simulink model "QBot2e_Particle_Filtering"  (Simulink 8.9)
settings: Solver=ode1  StartTime=0.0  StopTime=inf  FixedStep=0.01  RelTol=1e-3  EnableMultiTasking=on
InitFcn:
  | p=1:640; % pixels from left to right
  | 
  | Obtained_angles=(320-p).*(57/640)*pi./180;  % Kinect's horizontal FOV = 57 degrees
undefined symbols (not defined in the file): HIL, qc_get_step_size, Video3D
libraries: quarc_library x9, simulink x5
settings Model: Creator=drmadill  LastModifiedBy=User  SimulationMode=external  ExtModeTrigDuration=2
settings SolverCC: PositivePriorityOrder=on
settings OptimizationCC: ExpressionDepthLimit=2147483647  LifeSpan=auto
settings DebuggingCC: SolverPrmCheckMsg=warning
settings RTWCC: SystemTargetFile=quarc_linux_pi_3.tlc  TemplateMakefile=quarc_linux_pi_3_tmf  Description=QUARC Linux Raspberry Pi 3 Target
settings STFCustomTargetCC: TargetLibSuffix=.a  TargetPreCompLibLocation=C:\PROGRA~3\QUARC\lib\2019b\LINUX_~1\release  ConcurrentExecutionCompliant=on  SystemTargetFile=quarc_linux_pi_3.tlc
settings GRTTargetCC: TargetLibSuffix=.a  TargetPreCompLibLocation=C:\PROGRA~3\QUARC\lib\2017a\LICFC8~1\release  ParMdlRefBuildCompliant=off  CompOptLevelCompliant=off  GeneratePreprocessorConditionals=Use local settings  MatFileLogging=off  CPPClassGenCompliant=off  UseToolchainInfoCompliant=off  ExtMode=on  ExtModeMexFile=quarc_comm  ExtModeMexArgs='-w -d /tmp -uri %u'
settings ConfigComp: CovSFcnEnable=off

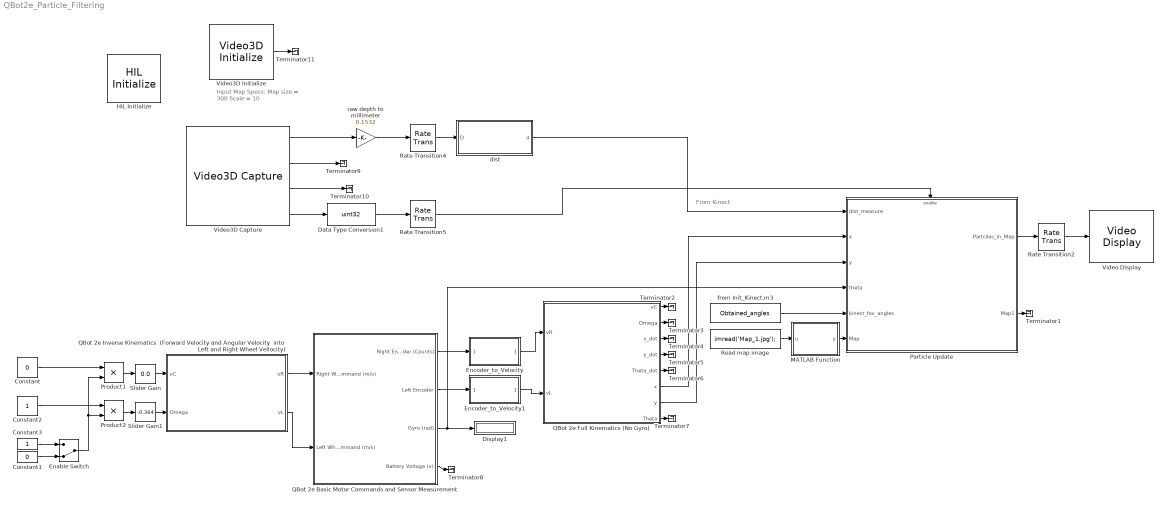
== system QBot2e_Particle_Filtering ==
  note: From Kinect
  note: Input Map Specs:
      | Map size = 300
      | Scale = 10
  Constant : Constant  Value=0
  Constant1 : Constant  Value=0
  Constant2 : Constant
  Constant3 : Constant
  Data Type Conversion1 : DataTypeConversion  OutDataTypeStr=uint32
  Display1 : Display
  Enable Switch : ManualSwitch  CurrentSetting=0
  Encoder_to_Velocity : Subsystem
  Encoder_to_Velocity1 : Subsystem
  HIL Initialize : quarc_library/Data Acquisition/Generic/Configuration/HIL Initialize  Priority=-99  object_name=HIL-1  board_type=qbot2e  board_number=0  board_options=pwm0_en=1;pwm0_pin=12;pwm1_en=1;pwm1_pin=13;  exclusive=off  active=off  hardware_clocks=[]  clock_modes=[]  initial_clock_frequencies=[]  set_clock_params_at_start=off  set_clock_params_at_switch_in=off  set_clock_frequencies_at_start=off  set_clock_frequencies_at_switch_in=off  analog_input_channels=[0:5]  analog_input_configurations=[]  analog_input_maximums=[16.5 3.3 3.3 3.3 3.3 3.3]  analog_input_minimums=[0 0 0 0 0 0]  set_analog_input_params_at_start=off  set_analog_input_params_at_switch_in=off  analog_output_channels=[]  analog_output_maximums=[]  analog_output_minimums=[]  initial_analog_outputs=[]  final_analog_outputs=[]  watchdog_analog_outputs=[]  set_analog_output_params_at_start=off  set_analog_output_params_at_switch_in=off  set_analog_outputs_at_start=off  set_analog_outputs_at_switch_in=off  set_analog_outputs_at_terminate=off  set_analog_outputs_at_switch_out=off  set_analog_outputs_on_watchdog=off  digital_input_channels=[28:58]  digital_output_channels=[28:31]  digital_output_configuration=[]  initial_digital_outputs=[0]  final_digital_outputs=[0]  watchdog_digital_outputs=[]  set_digital_output_params_at_start=off  set_digital_output_params_at_switch_in=off  set_digital_outputs_at_start=on  set_digital_outputs_at_switch_in=off  set_digital_outputs_at_terminate=on  set_digital_outputs_at_switch_out=off  set_digital_outputs_on_watchdog=off  encoder_channels=[0:1]  quadrature=[4]  encoder_filter_frequency=[]  initial_encoder_counts=[0]  set_encoder_params_at_start=on  set_encoder_params_at_switch_in=off  set_encoder_counts_at_start=on  set_encoder_counts_at_switch_in=off  pwm_channels=[0:1]  pwm_modes=0  pwm_frequency=100e6 / 4095  pwm_configuration=[0]  pwm_alignment=[0]  pwm_polarity=[1]  pwm_leading_deadband=[]  pwm_trailing_deadband=[]  initial_pwm_outputs=[0]  final_pwm_outputs=[0]  watchdog_pwm_outputs=[]  set_pwm_params_at_start=on  set_pwm_params_at_switch_in=off  set_pwm_outputs_at_start=on  set_pwm_outputs_at_switch_in=off  set_pwm_outputs_at_terminate=on  set_pwm_outputs_at_switch_out=off  set_pwm_outputs_on_watchdog=off  other_output_channels=[2000:2001 14000 16000]  initial_other_outputs=[0 0 0 7]  final_other_outputs=[0 0 0 7]  watchdog_other_outputs=[]  set_other_outputs_at_start=on  set_other_outputs_at_switch_in=off  set_other_outputs_at_terminate=on  set_other_outputs_at_switch_out=off  set_other_outputs_on_watchdog=off
  MATLAB Function : MATLAB Function  TreatAsAtomicUnit=on
  Particle Update : Subsystem  TreatAsAtomicUnit=on
  Product1 : Product  RndMeth=Zero
  Product2 : Product  RndMeth=Zero
  QBot 2e Basic Motor Commands and Sensor Measurement : Subsystem
  QBot 2e Full Kinematics (No Gyro) : Subsystem
  QBot 2e Inverse Kinematics  (Forward Velocity and Angular Velocity  into Left and Right Wheel Vellocity) : Subsystem
  Rate Transition2 : RateTransition
  Rate Transition4 : RateTransition
  Rate Transition5 : RateTransition
  Read map image : Constant  Value=imread('Map_1.jpg');
  Slider Gain : simulink/Math Operations/Slider Gain  gain=0.0  low=-1  high=1
  Slider Gain1 : simulink/Math Operations/Slider Gain  gain=-0.364  low=-0.7  high=0.7
  Terminator{1..11} (11 alike) : Terminator
  Video Display : quarc_library/Multimedia/Video Display  Tag=QBot2e_Particle_Filtering/Video Display  sample_time=-1  use_hardware=on
  Video3D Capture : quarc_library/Multimedia/Video3D Capture  object_name=Video3D-1  stream_type=Depth  stream_index=0  resolution=640 x 480  width=640  height=480  output_format=MATLAB greyscale (HxW)  data_type=uint16  sample_time=qc_get_step_size * ceil(0.033 / qc_get_step_size)  brightness_override=off  brightness=50.0  contrast_override=off  contrast=50.0  hue_override=off  hue=50.0  saturation_override=off  saturation=50.0  sharpness_override=off  sharpness=50.0  gamma_override=off  gamma=50.0  gain_override=off  gain=50.0  backlightcompensation_override=off  backlightcompensation=50.0  whitebalance_override=Automatic white balance  whitebalance=50.0  exposure_override=Automatic exposure  exposure=30.0  emitter=Enable laser emitter  preset=Do not set camera presets
  Video3D Initialize : quarc_library/Multimedia/Video3D Initialize  object_name=Video3D-1  source=Device  identifier=0  file=sample.bag  sample_time=qc_get_step_size * ceil(0.033 / qc_get_step_size)  active=on
  dist : MATLAB Function  TreatAsAtomicUnit=on
  from Init_Kinect.m3 : Constant  Value=Obtained_angles
  raw depth to millimeter : Gain  Gain=0.1532
  wires:
  Constant3/1 -> Enable Switch/1
  QBot 2e Basic Motor Commands and Sensor Measurement/1(Right Encoder (Counts)) -> Encoder_to_Velocity/1(Encoder)
  QBot 2e Basic Motor Commands and Sensor Measurement/2(Left Encoder) -> Encoder_to_Velocity1/1(Encoder)
  QBot 2e Basic Motor Commands and Sensor Measurement/3(Gyro (rad)) -> Display1/1, Particle Update/4(theta)
  QBot 2e Full Kinematics (No Gyro)/7(y) -> Particle Update/3(y)
  QBot 2e Full Kinematics (No Gyro)/6(x) -> Particle Update/2(x)
  Slider Gain/1 -> QBot 2e Inverse Kinematics  (Forward Velocity and Angular Velocity  into Left and Right Wheel Vellocity)/1(vC)
  Slider Gain1/1 -> QBot 2e Inverse Kinematics  (Forward Velocity and Angular Velocity  into Left and Right Wheel Vellocity)/2(Omega)
  from Init_Kinect.m3/1 -> Particle Update/5(kinect_fov_angles)
  dist/1(d) -> Particle Update/1(dist_measure)
  Particle Update/2(Map1) -> Terminator1/1
  QBot 2e Inverse Kinematics  (Forward Velocity and Angular Velocity  into Left and Right Wheel Vellocity)/1(vR) -> QBot 2e Basic Motor Commands and Sensor Measurement/1(Right Wheel Command (m/s))
  QBot 2e Inverse Kinematics  (Forward Velocity and Angular Velocity  into Left and Right Wheel Vellocity)/2(vL) -> QBot 2e Basic Motor Commands and Sensor Measurement/2(Left Wheel Command (m/s))
  Product1/1 -> Slider Gain/1
  Product2/1 -> Slider Gain1/1
  Enable Switch/1 -> Product2/2, Product1/2
  Constant/1 -> Product1/1
  Constant2/1 -> Product2/1
  Encoder_to_Velocity/1(Velocity) -> QBot 2e Full Kinematics (No Gyro)/1(vR)
  Encoder_to_Velocity1/1(Velocity) -> QBot 2e Full Kinematics (No Gyro)/2(vL)
  Constant1/1 -> Enable Switch/2
  QBot 2e Full Kinematics (No Gyro)/1(vC) -> Terminator2/1
  QBot 2e Full Kinematics (No Gyro)/2(Omega) -> Terminator3/1
  QBot 2e Full Kinematics (No Gyro)/3(x_dot) -> Terminator4/1
  QBot 2e Full Kinematics (No Gyro)/4(y_dot) -> Terminator5/1
  QBot 2e Full Kinematics (No Gyro)/5(Theta_dot) -> Terminator6/1
  QBot 2e Full Kinematics (No Gyro)/8(Theta) -> Terminator7/1
  Particle Update/1(Partciles_in_Map) -> Rate Transition2/1
  Rate Transition2/1 -> Video Display/1
  Read map image/1 -> MATLAB Function/1(u)
  MATLAB Function/1(y) -> Particle Update/6(Map)
  QBot 2e Basic Motor Commands and Sensor Measurement/4(Battery Voltage (v)) -> Terminator8/1
  Video3D Capture/2 -> Terminator9/1
  Video3D Capture/3 -> Terminator10/1
  Video3D Initialize/1 -> Terminator11/1
  Rate Transition5/1 -> Particle Update/Enable
  Video3D Capture/1 -> raw depth to millimeter/1
  Video3D Capture/4 -> Data Type Conversion1/1
  Data Type Conversion1/1 -> Rate Transition5/1
  Rate Transition4/1 -> dist/1(D)
  raw depth to millimeter/1 -> Rate Transition4/1

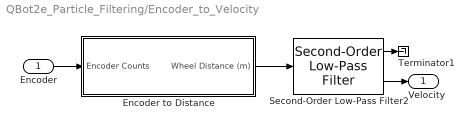
== system QBot2e_Particle_Filtering/Encoder_to_Velocity ==
  Encoder : Inport
  Encoder to Distance : Subsystem
  Second-Order Low-Pass Filter2 : quarc_library/Continuous/Second-Order Low-Pass Filter  params_source=Internal (dialog parameters)  input_width=10  input_zeta=1  input_init=0
  Terminator1 : Terminator
  Velocity : Outport
  wires:
  Second-Order Low-Pass Filter2/1 -> Terminator1/1
  Encoder to Distance/1(Wheel Distance (m)) -> Second-Order Low-Pass Filter2/1
  Encoder/1 -> Encoder to Distance/1(Encoder Counts)
  Second-Order Low-Pass Filter2/2 -> Velocity/1

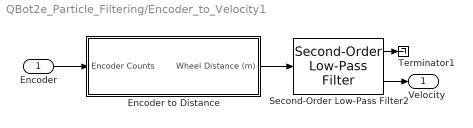
== system QBot2e_Particle_Filtering/Encoder_to_Velocity1 ==
  Encoder : Inport
  Encoder to Distance : Subsystem
  Second-Order Low-Pass Filter2 : quarc_library/Continuous/Second-Order Low-Pass Filter  params_source=Internal (dialog parameters)  input_width=10  input_zeta=1  input_init=0
  Terminator1 : Terminator
  Velocity : Outport
  wires:
  Second-Order Low-Pass Filter2/1 -> Terminator1/1
  Encoder to Distance/1(Wheel Distance (m)) -> Second-Order Low-Pass Filter2/1
  Encoder/1 -> Encoder to Distance/1(Encoder Counts)
  Second-Order Low-Pass Filter2/2 -> Velocity/1

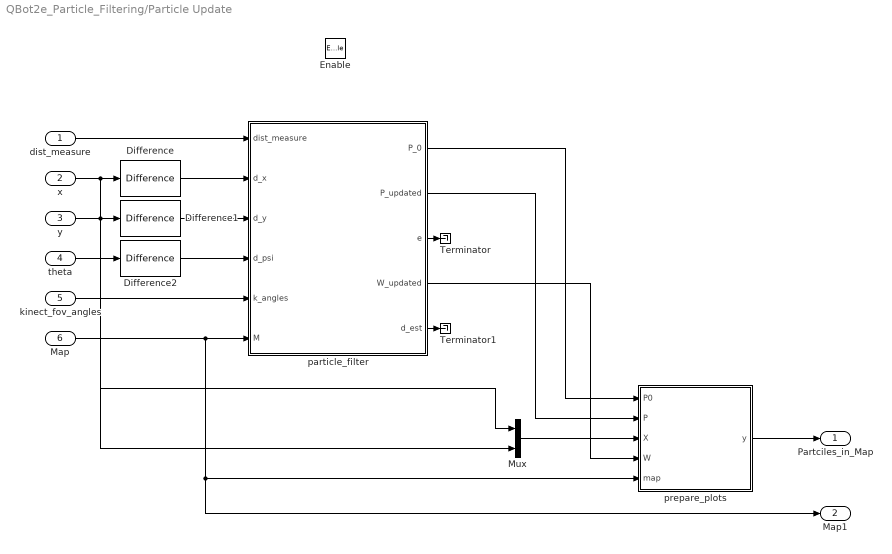
== system QBot2e_Particle_Filtering/Particle Update ==
  dist_measure : Inport
  x : Inport  Port=2
  y : Inport  Port=3
  theta : Inport  Port=4
  kinect_fov_angles : Inport  Port=5
  Map : Inport  Port=6
  Enable : EnablePort
  Difference : simulink/Discrete/Difference  ICPrevInput=0.0  OutMin=[]  OutMax=[]  OutDataType=fixdt(1, 16)  OutScaling=2^-10  DoSatur=off
  Difference1 : simulink/Discrete/Difference  ICPrevInput=0.0  OutMin=[]  OutMax=[]  OutDataType=fixdt(1, 16)  OutScaling=2^-10  DoSatur=off
  Difference2 : simulink/Discrete/Difference  ICPrevInput=0.0  OutMin=[]  OutMax=[]  OutDataType=fixdt(1, 16)  OutScaling=2^-10  DoSatur=off
  Mux : Mux  Inputs=2
  Terminator : Terminator
  Terminator1 : Terminator
  particle_filter : MATLAB Function  TreatAsAtomicUnit=on
  prepare_plots : MATLAB Function  TreatAsAtomicUnit=on
  Partciles_in_Map : Outport
  Map1 : Outport  Port=2
  wires:
  Map/1 -> Map1/1, prepare_plots/5(map), particle_filter/6(M)
  theta/1 -> Difference2/1
  y/1 -> Mux/2, Difference1/1
  x/1 -> Mux/1, Difference/1
  particle_filter/4(W_updated) -> prepare_plots/4(W)
  Difference2/1 -> particle_filter/4(d_psi)
  Difference1/1 -> particle_filter/3(d_y)
  Difference/1 -> particle_filter/2(d_x)
  Mux/1 -> prepare_plots/3(X)
  prepare_plots/1(y) -> Partciles_in_Map/1
  particle_filter/1(P_0) -> prepare_plots/1(P0)
  kinect_fov_angles/1 -> particle_filter/5(k_angles)
  particle_filter/2(P_updated) -> prepare_plots/2(P)
  dist_measure/1 -> particle_filter/1(dist_measure)
  particle_filter/3(e) -> Terminator/1
  particle_filter/5(d_est) -> Terminator1/1

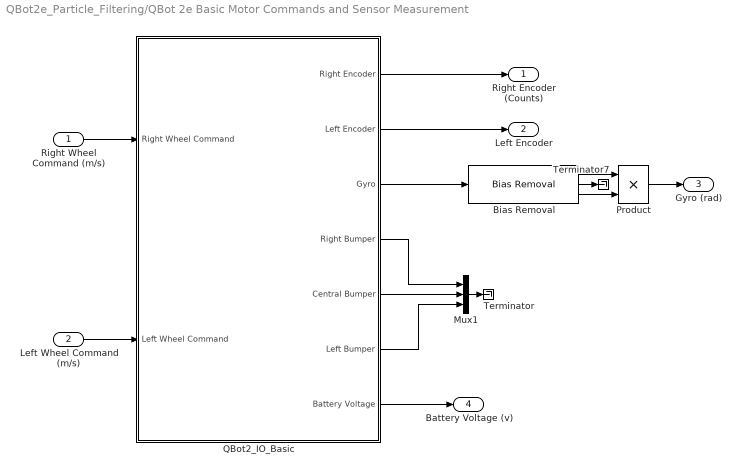
== system QBot2e_Particle_Filtering/QBot 2e Basic Motor Commands and Sensor Measurement ==
  Right Wheel Command (m/s) : Inport
  Left Wheel Command (m/s) : Inport  Port=2
  Bias Removal : quarc_library/Discrete/Bias Removal  start_time=3  end_time=4  switch_id=0  sample_time=qc_get_step_size
      settings: SourceProductName=QUARC Targets
  Mux1 : Mux  Inputs=3
  Product : Product  RndMeth=Zero
  QBot2_IO_Basic : Subsystem
  Terminator : Terminator
  Terminator7 : Terminator
  Right Encoder (Counts) : Outport
  Left Encoder : Outport  Port=2
  Gyro (rad) : Outport  Port=3
  Battery Voltage (v) : Outport  Port=4
  wires:
  QBot2_IO_Basic/4(Right Bumper) -> Mux1/1
  QBot2_IO_Basic/5(Central Bumper) -> Mux1/2
  QBot2_IO_Basic/6(Left Bumper) -> Mux1/3
  Right Wheel Command (m/s)/1 -> QBot2_IO_Basic/1(Right Wheel Command)
  Left Wheel Command (m/s)/1 -> QBot2_IO_Basic/2(Left Wheel Command)
  QBot2_IO_Basic/1(Right Encoder) -> Right Encoder (Counts)/1
  QBot2_IO_Basic/2(Left Encoder) -> Left Encoder/1
  QBot2_IO_Basic/7(Battery Voltage) -> Battery Voltage (v)/1
  Bias Removal/2 -> Terminator7/1
  Bias Removal/1 -> Product/1
  Bias Removal/3 -> Product/2
  Product/1 -> Gyro (rad)/1
  QBot2_IO_Basic/3(Gyro) -> Bias Removal/1
  Mux1/1 -> Terminator/1

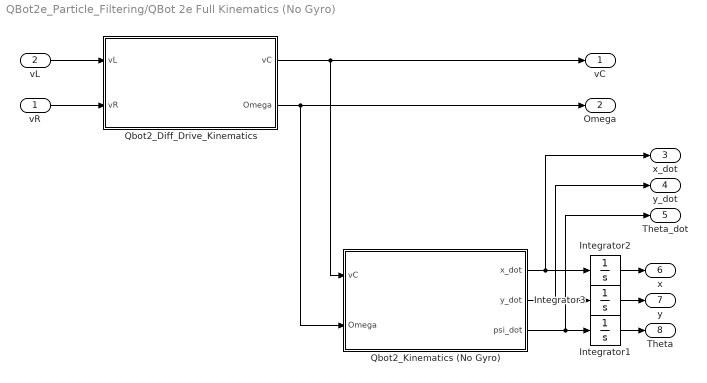
== system QBot2e_Particle_Filtering/QBot 2e Full Kinematics (No Gyro) ==
  vR : Inport
  vL : Inport  Port=2
  Integrator1 : Integrator
  Integrator2 : Integrator
  Integrator3 : Integrator
  Qbot2_Diff_Drive_Kinematics : Subsystem
  Qbot2_Kinematics (No Gyro) : Subsystem
  vC : Outport
  Omega : Outport  Port=2
  x_dot : Outport  Port=3
  y_dot : Outport  Port=4
  Theta_dot : Outport  Port=5
  x : Outport  Port=6
  y : Outport  Port=7
  Theta : Outport  Port=8
  wires:
  Qbot2_Diff_Drive_Kinematics/2(Omega) -> Omega/1, Qbot2_Kinematics (No Gyro)/2(Omega)
  Integrator3/1 -> y/1
  Integrator2/1 -> x/1
  vR/1 -> Qbot2_Diff_Drive_Kinematics/2(vR)
  vL/1 -> Qbot2_Diff_Drive_Kinematics/1(vL)
  Qbot2_Diff_Drive_Kinematics/1(vC) -> vC/1, Qbot2_Kinematics (No Gyro)/1(vC)
  Qbot2_Kinematics (No Gyro)/2(y_dot) -> Integrator3/1, y_dot/1
  Qbot2_Kinematics (No Gyro)/1(x_dot) -> Integrator2/1, x_dot/1
  Qbot2_Kinematics (No Gyro)/3(psi_dot) -> Integrator1/1, Theta_dot/1
  Integrator1/1 -> Theta/1

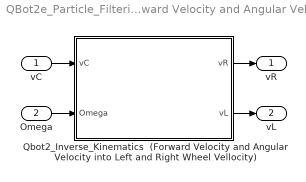
== system QBot2e_Particle_Filtering/QBot 2e Inverse Kinematics  (Forward Velocity and Angular Velocity  into Left and Right Wheel Vellocity) ==
  vC : Inport
  Omega : Inport  Port=2
  Qbot2_Inverse_Kinematics  (Forward Velocity and Angular Velocity into Left and Right Wheel Vellocity) : MATLAB Function  TreatAsAtomicUnit=on
  vR : Outport
  vL : Outport  Port=2
  wires:
  vC/1 -> Qbot2_Inverse_Kinematics  (Forward Velocity and Angular Velocity into Left and Right Wheel Vellocity)/1(vC)
  Qbot2_Inverse_Kinematics  (Forward Velocity and Angular Velocity into Left and Right Wheel Vellocity)/1(vR) -> vR/1
  Omega/1 -> Qbot2_Inverse_Kinematics  (Forward Velocity and Angular Velocity into Left and Right Wheel Vellocity)/2(Omega)
  Qbot2_Inverse_Kinematics  (Forward Velocity and Angular Velocity into Left and Right Wheel Vellocity)/2(vL) -> vL/1

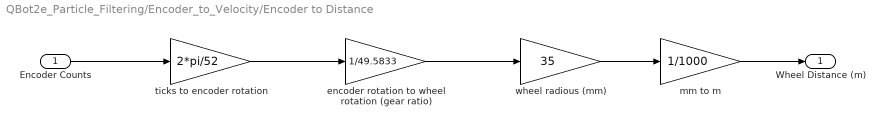
== system QBot2e_Particle_Filtering/Encoder_to_Velocity/Encoder to Distance ==
  Encoder Counts : Inport
  " encoder rotation to wheel rotation (gear ratio)" : Gain  Gain=1/49.5833
  mm to m : Gain  Gain=1/1000
  ticks to encoder rotation : Gain  Gain=2*pi/52
  wheel radious (mm) : Gain  Gain=35
  Wheel Distance (m) : Outport
  wires:
  Encoder Counts/1 -> ticks to encoder rotation/1
  ticks to encoder rotation/1 -> " encoder rotation to wheel rotation (gear ratio)"/1
  " encoder rotation to wheel rotation (gear ratio)"/1 -> wheel radious (mm)/1
  wheel radious (mm)/1 -> mm to m/1
  mm to m/1 -> Wheel Distance (m)/1

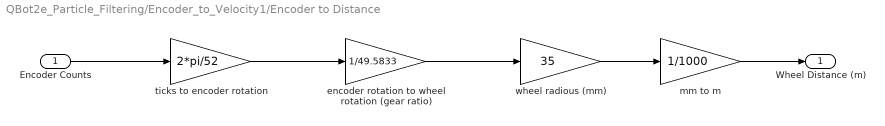
== system QBot2e_Particle_Filtering/Encoder_to_Velocity1/Encoder to Distance ==
  Encoder Counts : Inport
  " encoder rotation to wheel rotation (gear ratio)" : Gain  Gain=1/49.5833
  mm to m : Gain  Gain=1/1000
  ticks to encoder rotation : Gain  Gain=2*pi/52
  wheel radious (mm) : Gain  Gain=35
  Wheel Distance (m) : Outport
  wires:
  Encoder Counts/1 -> ticks to encoder rotation/1
  ticks to encoder rotation/1 -> " encoder rotation to wheel rotation (gear ratio)"/1
  " encoder rotation to wheel rotation (gear ratio)"/1 -> wheel radious (mm)/1
  wheel radious (mm)/1 -> mm to m/1
  mm to m/1 -> Wheel Distance (m)/1

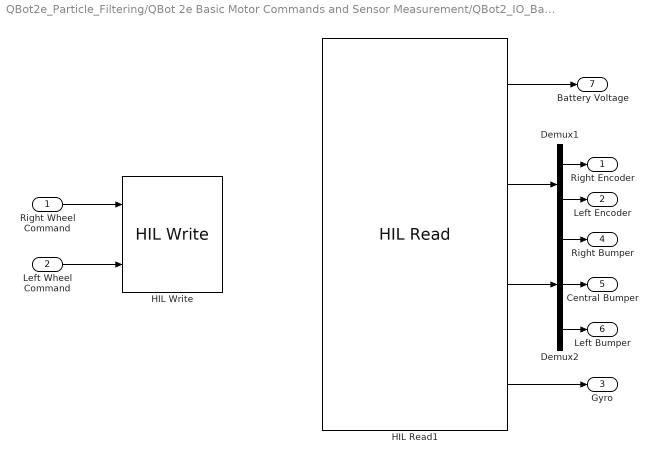
== system QBot2e_Particle_Filtering/QBot 2e Basic Motor Commands and Sensor Measurement/QBot2_IO_Basic ==
  Right Wheel Command : Inport
  Left Wheel Command : Inport  Port=2
  Demux1 : Demux  Outputs=2
  Demux2 : Demux  Outputs=3
  HIL Read1 : quarc_library/Data Acquisition/Generic/Immediate I//O/HIL Read  object_name=HIL-1  analog_channels=[0]  encoder_channels=[0:1]  digital_channels=[28:30]  other_channels=[1002]  sample_time=qc_get_step_size  active=on  vector_output=on  data_type_mode=Inherit via back propagation  encoder_data_type=double  digital_data_type=boolean
  HIL Write : quarc_library/Data Acquisition/Generic/Immediate I//O/HIL Write  object_name=HIL-1  analog_channels=[]  pwm_channels=[]  digital_channels=[]  other_channels=[2000:2001]  sample_time=-1  active=on  vector_input=off
  Right Encoder : Outport
  Left Encoder : Outport  Port=2
  Gyro : Outport  Port=3
  Right Bumper : Outport  Port=4
  Central Bumper : Outport  Port=5
  Left Bumper : Outport  Port=6
  Battery Voltage : Outport  Port=7
  wires:
  HIL Read1/1 -> Battery Voltage/1
  HIL Read1/3 -> Demux2/1
  HIL Read1/4 -> Gyro/1
  Demux1/1 -> Right Encoder/1
  Demux1/2 -> Left Encoder/1
  Right Wheel Command/1 -> HIL Write/1
  Left Wheel Command/1 -> HIL Write/2
  HIL Read1/2 -> Demux1/1
  Demux2/1 -> Right Bumper/1
  Demux2/2 -> Central Bumper/1
  Demux2/3 -> Left Bumper/1

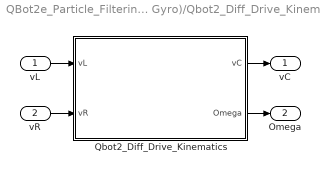
== system QBot2e_Particle_Filtering/QBot 2e Full Kinematics (No Gyro)/Qbot2_Diff_Drive_Kinematics ==
  vL : Inport
  vR : Inport  Port=2
  Qbot2_Diff_Drive_Kinematics : MATLAB Function  TreatAsAtomicUnit=on
  vC : Outport
  Omega : Outport  Port=2
  wires:
  Qbot2_Diff_Drive_Kinematics/2(Omega) -> Omega/1
  vR/1 -> Qbot2_Diff_Drive_Kinematics/2(vR)
  Qbot2_Diff_Drive_Kinematics/1(vC) -> vC/1
  vL/1 -> Qbot2_Diff_Drive_Kinematics/1(vL)

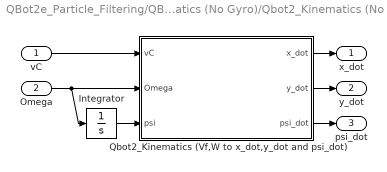
== system QBot2e_Particle_Filtering/QBot 2e Full Kinematics (No Gyro)/Qbot2_Kinematics (No Gyro) ==
  vC : Inport
  Omega : Inport  Port=2
  Integrator : Integrator
  Qbot2_Kinematics (Vf,W to x_dot,y_dot and psi_dot) : MATLAB Function  TreatAsAtomicUnit=on
  x_dot : Outport
  y_dot : Outport  Port=2
  psi_dot : Outport  Port=3
  wires:
  Qbot2_Kinematics (Vf,W to x_dot,y_dot and psi_dot)/2(y_dot) -> y_dot/1
  Omega/1 -> Qbot2_Kinematics (Vf,W to x_dot,y_dot and psi_dot)/2(Omega), Integrator/1
  Qbot2_Kinematics (Vf,W to x_dot,y_dot and psi_dot)/1(x_dot) -> x_dot/1
  vC/1 -> Qbot2_Kinematics (Vf,W to x_dot,y_dot and psi_dot)/1(vC)
  Integrator/1 -> Qbot2_Kinematics (Vf,W to x_dot,y_dot and psi_dot)/3(psi)
  Qbot2_Kinematics (Vf,W to x_dot,y_dot and psi_dot)/3(psi_dot) -> psi_dot/1

== matlab function dist ==
  data: D input double; d output double
function d  = fcn(D)
%#codegen

    LINE=240;

    d=double(D(LINE,:)/1000)'; % into meter
    

    
  %alpha= -(LINE-240)*43*pi/180/480; % Vertical FOV
  %z=  tan(alpha)*L.*ones(640,1);

== matlab function Particle Update/particle_filter ==
  data: P_0 output double; dist_measure input double; P_updated output double; d_x input double; d_y input double; d_psi input double; k_angles input double; M input double; e output double; W_updated output double; d_est output double
function [P_0, P_updated,e,W_updated, d_est] = fcn(dist_measure,d_x,d_y,d_psi,k_angles,M)
%#codegen

%particle_sense(x,y,psi,k_angles,M);
N=100;
%no_Iterations=1;

sigma_measure=0.4;
sigma_move=0.05;
sigma_rotate=0.05;

%ah: initialize Particles if empty
persistent P;
persistent P0;
persistent W;

if isempty(W);
   W=ones(N,1)/N;
end

if isempty(P)
    P=zeros(N,3);
    for i=1:N
        p_x=rand()*3-1.5; % [-1.5 1.5] centre around 0 (can fit in a 90x90 map scaled 4.5)
        p_y=rand()*3-1.5; % [-1.5 1.5] centre around 0  (can fit in a 90x90 map scaled 4.5)
        p_psi=rand()*2*pi;
        P(i,:)=[p_x p_y p_psi];
    end
 
end


if isempty(P0)
    P0=P;
end

N=length(P);
P1=zeros(N,3);
%P_updated=P1;
e=zeros(N,1);


d_resampled=resample_data(dist_measure);
d_est=zeros(length(P),length(d_resampled));


%for k=1:no_Iterations
    
   for i=1:N
        % ah: move the particles the same way that robo moves!

        P(i,1)=P(i,1)+d_x+cos(P(i,3))*sigma_move*randn(1);
        P(i,2)=P(i,2)+d_y+sin(P(i,3))*sigma_move*randn(1);
        P(i,3)=P(i,3)+d_psi+sigma_rotate*randn(1);
        
        %W(i)=P(i).measurementProb(Z);
        
        % ah: estimate dist if P(i,:) was the correct representation of the
        % robot
               
        d_est(i,:)=particle_sense(P(i,1),P(i,2),P(i,3),k_angles,M);
        e(i)=(sqrt((d_est(i,:)-d_resampled')*(d_est(i,:)-d_resampled')'))/length(d_est);
       
    end

    %Update Weight based on the Proposed Gaussian Distribution
    W=(1/(sqrt((2*pi))*sigma_measure)).*(exp(-0.5*e.^2/((sigma_measure^2))));
    n=sum(W);
    W=W/n; %normalized weight array

    %Update the predictions
    %[Wmax ImW]=max(W);
    
    %Randomly draw particles from the current particles with high weights
    
    
    beta=0;
    index=randi(N-1);
    [W_max, ImW]=max(W);
    
    for i=1:N
        offSet=rand(1)*2*W_max;
        beta=beta+offSet(1);
        while(beta>W(index))
            beta=beta-W(index);
            index=index+1;
            if(index==N)
                index=index-N+1;
            end
        end
        %index represent a particle with a weight higher than randomly
        %manipulated beta - in general we keep the high weights over time
        P1(i,:)=P(index,:);
    end
     P=P1;
    
       
   
    P_updated=P;
    P_0=P0;
    W_updated=W;
  
end

== matlab function Particle Update/prepare_plots ==
  data: P0 input double; P input double; y output uint8 size=[301 301 3]; X input double; W input double; map input uint8 size=[301 301]
function y = fcn(P0,P,X,W,map)
%#codegen

S=300;
scale = 10;



P(P>2.5)=2.5;
P(P<-2.5)=-2.5;

P0(P0>2.5)=5;
P0(P0<-2.5)=-2.5;

X(X>5)=5;
X(X<-5)=-5;

M=uint8(255*ones(S+1,S+1,3));

for i=1:S
    for j=1:S
        M(i,j,1)=map(i,j);
    end
end


for i=1:length(P0)
M(round(P0(i,1)*scale)+S/2+1,round(P0(i,2)*scale)+S/2+1,2)=230; % matrix indices start from 1 + centre the data 
M(round(P0(i,1)*scale)+S/2+1,round(P0(i,2)*scale)+S/2+1,1)=100; % matrix indices start from 1 + centre the data 
M(round(P0(i,1)*scale)+S/2+1,round(P0(i,2)*scale)+S/2+1,3)=100; % matrix indices start from 1 + centre the data 

end


for i=1:length(P)
M(round(P(i,1)*scale)+S/2+1,round(P(i,2)*scale)+S/2+1,1)=120-round(100*W(i)); % matrix indices start from 1 + centre the data 
M(round(P(i,1)*scale)+S/2+1,round(P(i,2)*scale)+S/2+1,2)=120-round(100*W(i)); % matrix indices start from 1 + centre the data 
M(round(P(i,1)*scale)+S/2+1,round(P(i,2)*scale)+S/2+1,3)=0; % matrix indices start from 1 + centre the data 
end



M(round(X(1)*scale)+S/2+1,round(X(2)*scale)+S/2+1,1)=0; % matrix indices start from 1 + centre the data 
M(round(X(1)*scale)+S/2+1,round(X(2)*scale)+S/2+1,2)=0; % matrix indices start from 1 + centre the data 
M(round(X(1)*scale)+S/2+1,round(X(2)*scale)+S/2+1,3)=0; % matrix indices start from 1 + centre the data 



y=M;

%y=map;

== matlab function QBot 2e Full Kinematics (No Gyro)/Qbot2_Diff_Drive_Kinematics/Qbot2_Diff_Drive_Kinematics ==
  data: vL input double; vC output double; vR input double; Omega output double
function [vC,Omega] = fcn(vL,vR)
%#codegen

d= 0.235;

vC=0.5*(vL+vR);
Omega=(1/d)*(vR-vL);

== matlab function QBot 2e Full Kinematics (No Gyro)/Qbot2_Kinematics (No Gyro)/Qbot2_Kinematics (Vf,W to x_dot,y_dot and psi_dot) ==
  data: vC input double; x_dot output double; Omega input double; y_dot output double; psi input double; psi_dot output double
function [x_dot,y_dot,psi_dot] = fcn(vC,Omega,psi)
%#codegen


x_dot=cos(psi)*vC;
y_dot=sin(psi)*vC;
psi_dot= Omega;

== matlab function MATLAB Function ==
  data: u input double; y output double
function y = fcn(u)
y = u(:,:,3);

== matlab function QBot 2e Inverse Kinematics (Forward Velocity and Angular Velocity into Left and Right Wheel Vellocity)/Qbot2_Inverse_Kinematics (Forward Velocity and Angular Velocity into Left and Right Wheel Vellocity) ==
  data: vR output double; vL output double; vC input double; Omega input double
function [vR,vL] = fcn(vC , Omega)
%#codegen

d=0.235; 
% Eqn Based on the eqn 4.52 (W is the angular velocity)

vR = vC + Omega*d/2;
vL= vC - Omega*d/2;
